simulink model "TestaBlocosUteis1"  (R2020b)
settings: Solver=FixedStepDiscrete  StartTime=0.0  StopTime=15  FixedStep=1  RelTol=1e-3
InitFcn:
  | CarregaTabelas
  | Ts=10;
  | FreqIni=40;
  | PChegadaIni=20;
  | PSucIni=100;
  | VazaoIni=230;
  | FreqENG=55;
  | PMonENG=35;
values from neighbouring files (symbols this model uses):
  BTP = readtable('DoBTP.xlsx')    [CarregaTabelas.m]
  FxPercent = readtable('DP-Faixas.xlsx')    [CarregaTabelas.m]    (also in ProtecaoDinamica.m)
  ProtecaoFixa = readtable('FixedProtections.xlsx')    [CarregaTabelas.m]
  TabRestricoesDinamicas = readtable('DP.xlsx')    [CarregaTabelas.m]
  TabSimulador = LeConverteNomes('DoSimulador.xlsx')    [CarregaTabelas.m]
settings Model: Creator=leize  LastModifiedBy=leize

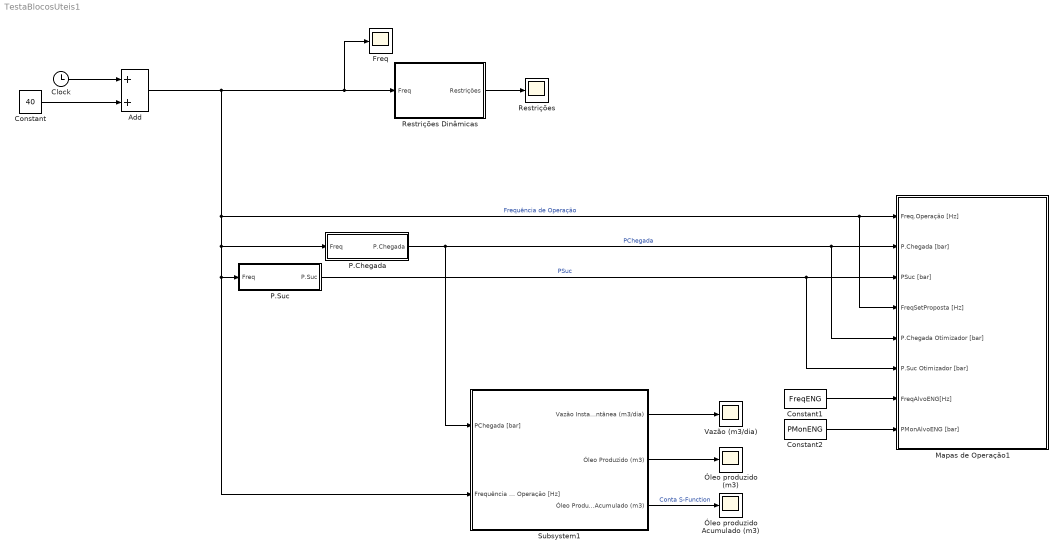
== system TestaBlocosUteis1 ==
  Add : Sum
  Clock : Clock
  Constant : Constant  Value=40
  Constant1 : Constant  Value=FreqENG
  Constant2 : Constant  Value=PMonENG
  Freq : Scope
  Mapas de Operação1 : Subsystem  mask{PlotaMapas=1, HabilitaRastro=1, Tsim=TabSimulador, BTP=BTP, FreqIni=FreqIni, PChegadaIni=PChegadaIni, PSucIni=PSucIni, FreqAlvoIni=FreqENG, PMonAlvoIni=PMonENG}
      mask prompts: PlotaMapas "Plotar Mapas (1/0)?"; HabilitaRastro "Habilita Rastro do Plot (1/0)?"; Tsim "Tabela do Simulador"; BTP "Tabela BTP"; FreqIni "Frequencia Inicial [Hz]"; PChegadaIni "PChegada Inicial [bar]"; PSucIni "Pressao de Succao Inicial [bar]"; FreqAlvoIni "Frequencia ALVO Inicial [Hz]"; PMonAlvoIni "PChegada ALVO [bar]"
      mask DialogControl DescTextVar Prompt: MAPAS DE OPERAÇÃO
      mask DialogControl ParameterGroupVar Prompt: Tabelas Petrobras e configurações dos Mapas de Operação
      mask DialogControl ParameterGroupVar_copy Prompt: Dados do Processo
      mask DialogControl ParameterGroupVar_copy_copy_copy Prompt: Dados Engenharia (Alvos)
  P.Chegada : Subsystem
  P.Suc : Subsystem
  Restrições : Scope
  Restrições Dinâmicas : Subsystem
  Subsystem1 : Subsystem  mask{TabSimulador=TabSimulador, DeltaT=Ts, QIni=VazaoIni}
      mask prompts: TabSimulador "Tabela do Simulador"; DeltaT "Periodo de amostragem (s)"; QIni "Vazao Inicial (m3/dia)"
  Vazão (m3/dia) : Scope
  Óleo produzido (m3) : Scope
  Óleo produzido Acumulado (m3) : Scope
  wires:
  Constant/1 -> Add/2
  Clock/1 -> Add/1
  Add/1 -> Restrições Dinâmicas/1(Freq), Freq/1, Mapas de Operação1/4(FreqSetProposta [Hz]), Mapas de Operação1/1(Freq.Operação [Hz]), Subsystem1/2(Frequência de Operação [Hz]), P.Suc/1(Freq), P.Chegada/1(Freq)  "Frequência de Operação"
  Restrições Dinâmicas/1(Restrições) -> Restrições/1
  P.Chegada/1(P.Chegada) -> Subsystem1/1(PChegada [bar]), Mapas de Operação1/5(P.Chegada Otimizador [bar]), Mapas de Operação1/2(P.Chegada [bar])  "PChegada"
  Subsystem1/2("Óleo Produzido (m3) ") -> Óleo produzido (m3)/1
  Subsystem1/3(Óleo Produzido Acumulado (m3)) -> Óleo produzido Acumulado (m3)/1  "Conta S-Function"
  P.Suc/1(P.Suc) -> Mapas de Operação1/6(P.Suc Otimizador [bar]), Mapas de Operação1/3(PSuc [bar])  "PSuc"
  Constant1/1 -> Mapas de Operação1/7(FreqAlvoENG[Hz])
  Constant2/1 -> Mapas de Operação1/8(PMonAlvoENG [bar])
  Subsystem1/1(Vazão Instantânea (m3/dia)) -> Vazão (m3/dia)/1

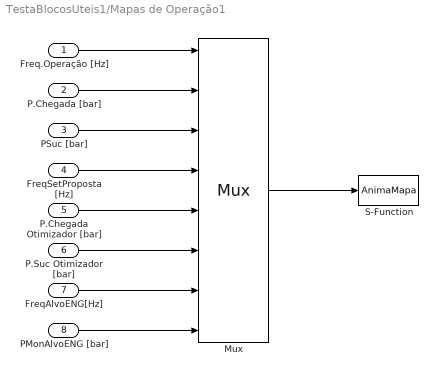
== system TestaBlocosUteis1/Mapas de Operação1 ==
  Freq.Operação [Hz] : Inport
  P.Chegada [bar] : Inport  Port=2
  PSuc [bar] : Inport  Port=3
  FreqSetProposta [Hz] : Inport  Port=4
  P.Chegada Otimizador [bar] : Inport  Port=5
  P.Suc Otimizador [bar] : Inport  Port=6
  FreqAlvoENG[Hz] : Inport  Port=7
  PMonAlvoENG [bar] : Inport  Port=8
  Mux : Mux  Inputs=8
  S-Function : S-Function  FunctionName=AnimaMapa  Parameters=PlotaMapas,Tsim,BTP,FreqIni, PChegadaIni,PSucIni,FreqAlvoIni,PMonAlvoIni,HabilitaRastro  SFunctionDeploymentMode=off  EnableBusSupport=off
  wires:
  Freq.Operação [Hz]/1 -> Mux/1
  Mux/1 -> S-Function/1
  P.Chegada [bar]/1 -> Mux/2
  PSuc [bar]/1 -> Mux/3
  P.Chegada Otimizador [bar]/1 -> Mux/5
  P.Suc Otimizador [bar]/1 -> Mux/6
  FreqAlvoENG[Hz]/1 -> Mux/7
  PMonAlvoENG [bar]/1 -> Mux/8
  FreqSetProposta [Hz]/1 -> Mux/4

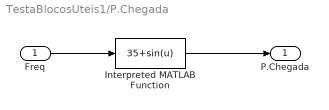
== system TestaBlocosUteis1/P.Chegada ==
  Freq : Inport
  Interpreted MATLAB Function : MATLABFcn  MATLABFcn=35+sin(u)
  P.Chegada : Outport
  wires:
  Interpreted MATLAB Function/1 -> P.Chegada/1
  Freq/1 -> Interpreted MATLAB Function/1

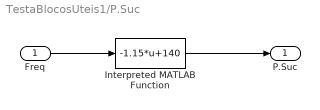
== system TestaBlocosUteis1/P.Suc ==
  Freq : Inport
  Interpreted MATLAB Function : MATLABFcn  MATLABFcn=-1.15*u+140
  P.Suc : Outport
  wires:
  Freq/1 -> Interpreted MATLAB Function/1
  Interpreted MATLAB Function/1 -> P.Suc/1

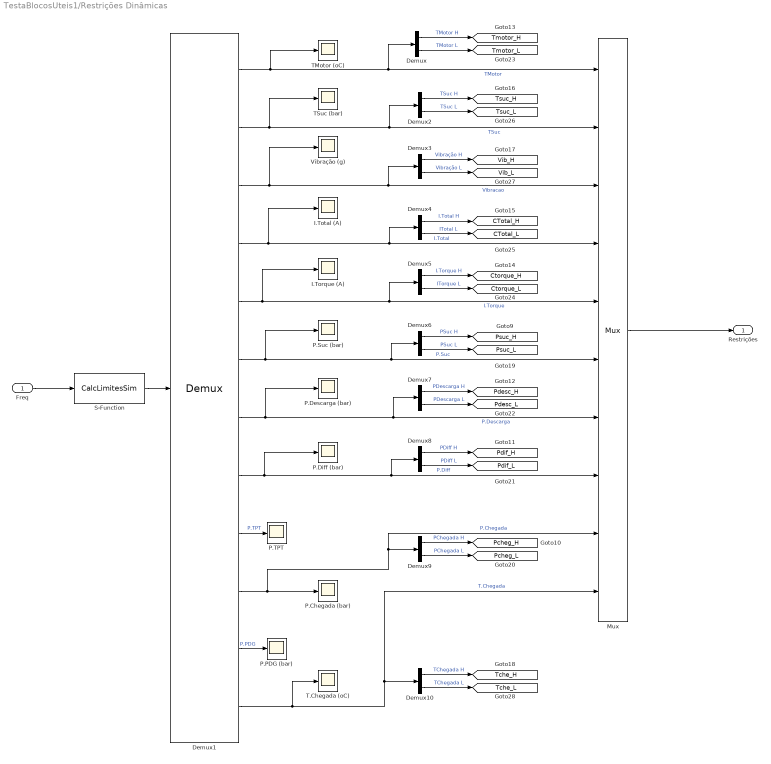
== system TestaBlocosUteis1/Restrições Dinâmicas ==
  Freq : Inport
  Demux{,2..10} (10 alike) : Demux  Outputs=2
  Demux1 : Demux  Outputs=[ 2 2 2 2 2 2 2 2 2 2 2 2]
  I.Torque (A) : Scope
  I.Total (A) : Scope
  Mux : Mux  Inputs=[ 2 2 2 2 2 2 2 2 2 2]
  P.Chegada (bar) : Scope
  P.Descarga (bar) : Scope
  P.Diff (bar) : Scope
  P.PDG (bar) : Scope
  P.Suc (bar) : Scope
  P.TPT : Scope
  S-Function : S-Function  FunctionName=CalcLimitesSim  Parameters=FreqIni,TabSimulador,BTP,TabRestricoesDinamicas,FxPercent,ProtecaoFixa  SFunctionDeploymentMode=off  EnableBusSupport=off
  T.Chegada (oC) : Scope
  TMotor (oC) : Scope
  TSuc (bar) : Scope
  Vibração (g) : Scope
  Restrições : Outport
  tag scope: CTotal_H=global, CTotal_L=global, Ctorque_H=global, Ctorque_L=global, Pcheg_H=global, Pcheg_L=global, Pdesc_H=global, Pdesc_L=global, Pdif_H=global, Pdif_L=global, Psuc_H=global, Psuc_L=global, Tche_H=global, Tche_L=global, Tmotor_H=global, Tmotor_L=global, Tsuc_H=global, Tsuc_L=global, Vib_H=global, Vib_L=global
  wires:
  Demux1/3 -> Demux3/1, Mux/3, Vibração (g)/1  "Vibracao"
  Demux1/7 -> Demux7/1, Mux/7, P.Descarga (bar)/1  "P.Descarga"
  Demux1/12 -> Demux10/1, Mux/10, T.Chegada (oC)/1  "T.Chegada"
  Demux1/6 -> Demux6/1, Mux/6, P.Suc (bar)/1  "P.Suc"
  Demux1/10 -> Demux9/1, Mux/9, P.Chegada (bar)/1  "P.Chegada"
  Demux1/9 -> P.TPT/1  "P.TPT"
  Demux1/8 -> Demux8/1, Mux/8, P.Diff (bar)/1  "P.Diff"
  Freq/1 -> S-Function/1
  S-Function/1 -> Demux1/1
  Demux1/11 -> P.PDG (bar)/1  "P.PDG"
  Demux1/1 -> TMotor (oC)/1, Demux/1, Mux/1  "TMotor"
  Demux1/2 -> Demux2/1, Mux/2, TSuc (bar)/1  "TSuc"
  Demux1/5 -> Demux5/1, Mux/5, I.Torque (A)/1  "I.Torque"
  Demux1/4 -> Demux4/1, Mux/4, I.Total (A)/1  "I.Total"
  Mux/1 -> Restrições/1
  Demux/2 -> [Tmotor_L]  "TMotor L"
  Demux/1 -> [Tmotor_H]  "TMotor H"
  Demux6/1 -> [Psuc_H]  "PSuc H"
  Demux9/1 -> [Pcheg_H]  "PChegada H"
  Demux8/1 -> [Pdif_H]  "PDiff H"
  Demux7/1 -> [Pdesc_H]  "PDescarga H"
  Demux5/1 -> [Ctorque_H]  "I.Torque H"
  Demux4/1 -> [CTotal_H]  "I.Total H"
  Demux2/1 -> [Tsuc_H]  "TSuc H"
  Demux3/1 -> [Vib_H]  "Vibração H"
  Demux10/1 -> [Tche_H]  "TChegada H"
  Demux6/2 -> [Psuc_L]  "PSuc L"
  Demux9/2 -> [Pcheg_L]  "PChegada L"
  Demux8/2 -> [Pdif_L]  "PDiff L"
  Demux7/2 -> [Pdesc_L]  "PDescarga L"
  Demux4/2 -> [CTotal_L]  "ITotal L"
  Demux2/2 -> [Tsuc_L]  "TSuc L"
  Demux3/2 -> [Vib_L]  "Vibração L"
  Demux10/2 -> [Tche_L]  "TChegada L"
  Demux5/2 -> [Ctorque_L]  "ITorque L"

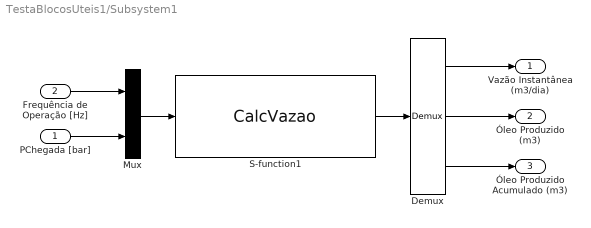
== system TestaBlocosUteis1/Subsystem1 ==
  PChegada [bar] : Inport
  Frequência de Operação [Hz] : Inport  Port=2
  Demux : Demux  Outputs=3
  Mux : Mux  Inputs=2
  S-function1 : S-Function  FunctionName=CalcVazao  Parameters=TabSimulador,DeltaT,QIni  SFunctionDeploymentMode=off  EnableBusSupport=off
  Vazão Instantânea (m3/dia) : Outport
  "Óleo Produzido (m3) " : Outport  Port=2
  Óleo Produzido Acumulado (m3) : Outport  Port=3
  wires:
  PChegada [bar]/1 -> Mux/2
  Frequência de Operação [Hz]/1 -> Mux/1
  Mux/1 -> S-function1/1
  S-function1/1 -> Demux/1
  Demux/2 -> "Óleo Produzido (m3) "/1
  Demux/3 -> Óleo Produzido Acumulado (m3)/1
  Demux/1 -> Vazão Instantânea (m3/dia)/1
